simulink model "TV_2017_HIL"  (R2016a)
settings: Solver=ode1  StartTime=0.0  StopTime=600  FixedStep=0.001  RelTol=1e-3
PreLoadFcn:
  | HIL_parameters
values from neighbouring files (symbols this model uses):
  battery_voltage = single(530)    [HIL_parameters.m]    (also in HIL_parameters_2018.m; TV_2017_parameters.m; TV_2017_parameters_VD.m)
  car_params = Simulink_Car_params    [HIL_parameters.m]    (also in HIL_parameters_2018.m; TV_2017_parameters.m; TV_2017_parameters_VD.m)
  i_Diff = 16    [HIL_parameters.m]    (also in HIL_parameters_2018.m; TV_2017_parameters.m)
  Kp = 1    [HIL_parameters.m]    (also in HIL_parameters_2018.m; TV_2017_parameters.m; TV_2017_parameters_VD.m)
  motor_data = struct    [HIL_parameters.m]    (also in HIL_parameters_2018.m; TV_2017_parameters.m)
  settings = Simulink_Settings    [HIL_parameters.m]    (also in HIL_parameters_2018.m; TV_2017_parameters.m; TV_2017_parameters_VD.m)
  SpdC_BCC = 0    [HIL_parameters.m]    (also in HIL_parameters_2018.m; TV_2017_parameters.m; TV_2017_parameters_VD.m)
  Speed_Neg_sat = -21    [HIL_parameters.m]    (also in HIL_parameters_2018.m; TV_2017_parameters.m; TV_2017_parameters_VD.m)
  Speed_Pos_sat = 21    [HIL_parameters.m]    (also in HIL_parameters_2018.m; TV_2017_parameters.m; TV_2017_parameters_VD.m)
  SteeringAngleFL = [-23.80 -22.65 -21.50 -20.34 -19.18 -18.03 -16.86 -15.70 -14.53 -13.35 -12.18 -10.99 -9.80 -8.61 -7.40 -6.19 -4.97 -3.75 -2.51 -1.26 0 1.27 2.56 3.85 5.17 6.50 7.84 9.21 10.59 12.00 13.42 14.88 16.36 17.87 19.41 20.99 22.61 24.26 25.97 27.73 29.54]    [CarSetupAnalysis2018.m]    (also in HIL_parameters_2018.m; TV_2017_parameters.m; TV_2017_parameters_VD.m = [-24.129 -22.950 -21.772 -20.593 -19.413 -18.232 -17.050 -15)
  SteeringAngleFR = [-29.54 -27.73 -25.97 -24.26 -22.61 -20.99 -19.41 -17.87 -16.36 -14.88 -13.42 -12.00 -10.59 -9.21 -7.84 -6.50 -5.17 -3.85 -2.56 -1.27 0 1.26 2.51 3.75 4.97 6.19 7.40 8.61 9.80 10.99 12.18 13.35 14.53 15.70 16.86 18.03 19.18 20.34 21.50 22.65 23.80]    [CarSetupAnalysis2018.m]    (also in HIL_parameters_2018.m; TV_2017_parameters.m; TV_2017_parameters_VD.m = [-29.3050 -27.5340 -25.8140 -24.1410 -22.5110 -20.9180 -19.3)
  SteeringWhAngle = [-105 -99.75 -94.5 -89.25 -84 -78.75 -73.5 -68.25 -63 -57.75 -52.5 -47.25 -42 -36.75 -31.5 -26.25 -21.0 -15.75 -10.5 -5.25 0.0 5.25 10.50 15.75 21.00 26.25 31.50 36.75 42.00 47.25 52.50 57.75  63.00 68.25 73.50 78.75 84.00 89.25 94.50 99.75 105.00]    [TV_2017_parameters_VD.m]
  Tn_n = 0    [HIL_parameters.m]    (also in HIL_parameters_2018.m; TV_2017_parameters.m; TV_2017_parameters_VD.m)
  Use_Joystick = 1    [HIL_parameters.m]    (also in HIL_parameters_2018.m; TV_2017_parameters.m; TV_2017_parameters_VD.m)
undefined symbols (not defined in the file or in its folder): canChannel, TC_Decr_Gas, TC_Derivative, TC_Incr_Gas, TC_On, TC_Relay_Off, TC_Relay_On
libraries: CarMaker4SL x314, canmsglib x48, simulink_extras x48, simulink x41, canlib x39, powerlib_meascontrol x2, sldrtlib x1
(part 9 of 9)

== system TV_2017_HIL/CarMaker/IPG Vehicle3/CarAndTrailer/Forces/Tires/TireRR ==
  note: Insert your tire model here.
  Sync_In : Inport
  Load : Inport  Port=2
  vxtrans : Inport  Port=3
  vytrans : Inport  Port=4
  Rim_rotv : Inport  Port=5
  Rim_turnv : Inport  Port=6
  InclinAngle : Inport  Port=7
  muRoad : Inport  Port=8
  Ground{1..11} (11 alike) : Ground
  Terminator{,1..6,12} (8 alike) : Terminator
  Slp : Outport
  Alpha : Outport  Port=2
  TurnSlp : Outport  Port=3
  rBelt_eff : Outport  Port=4
  vBelt : Outport  Port=5
  LongFrc : Outport  Port=6
  SideFrc : Outport  Port=7
  LoadFrc : Outport  Port=8
  OverturnTrq : Outport  Port=9
  RollResist : Outport  Port=10
  AlignTrq : Outport  Port=11
  wires:
  Ground11/1 -> vBelt/1
  Ground10/1 -> rBelt_eff/1
  Ground9/1 -> TurnSlp/1
  Rim_turnv/1 -> Terminator6/1
  Sync_In/1 -> Terminator12/1
  Ground2/1 -> Alpha/1
  Ground3/1 -> LongFrc/1
  Ground4/1 -> SideFrc/1
  Ground5/1 -> OverturnTrq/1
  vxtrans/1 -> Terminator1/1
  vytrans/1 -> Terminator2/1
  Rim_rotv/1 -> Terminator3/1
  InclinAngle/1 -> Terminator4/1
  muRoad/1 -> Terminator5/1
  Load/1 -> Terminator/1
  Ground1/1 -> Slp/1
  Ground6/1 -> LoadFrc/1
  Ground7/1 -> RollResist/1
  Ground8/1 -> AlignTrq/1

== system TV_2017_HIL/CarMaker/IPG Vehicle3/CarAndTrailer/Forces/Vehicle Forces/Aero R18 prelim ==
  car Aero ApproachVel_1 x : Inport
  car Aero ApproachVel_1 y : Inport  Port=2
  car Aero ApproachVel_1 z : Inport  Port=3
  car Aero tau_1 : Inport  Port=4
  car Aero PoA_1 x : Inport  Port=5
  car Aero PoA_1 y : Inport  Port=6
  car Aero PoA_1 z : Inport  Port=7
  car Aero Frc_1 x : Inport  Port=8
  car Aero Frc_1 y : Inport  Port=9
  car Aero Frc_1 z : Inport  Port=10
  car Aero Trq_1 x : Inport  Port=11
  car Aero Trq_1 y : Inport  Port=12
  car Aero Trq_1 z : Inport  Port=13
  Coefficients : Subsystem
  Constant : Constant  Value=0
  Drag & DF : Scope  NumInputPorts=2
  MATLAB Function : MATLAB Function  TreatAsAtomicUnit=on
  Pitch moment : Scope
  Rad2Deg : simulink_extras/Transformations/Radians to Degrees
  Rad2Deg1 : simulink_extras/Transformations/Radians to Degrees
  Rad2Deg2 : simulink_extras/Transformations/Radians to Degrees
  Read CM Dict : CarMaker4SL/Read CM Dict  xname=Car.Roll  xsync=off
  Read CM Dict1 : CarMaker4SL/Read CM Dict  xname=Car.Pitch  xsync=off
  Read CM Dict2 : CarMaker4SL/Read CM Dict  xname=Car.TrackRadius  xsync=off
  Scope : Scope  Commented=on  NumInputPorts=2
  Terminator{,1..5} (6 alike) : Terminator
  Yaw moment : Scope
  car Aero ApproachVel_1 x_R18 : Outport
  car Aero ApproachVel_1 y_R18 : Outport  Port=2
  car Aero ApproachVel_1 z_R18 : Outport  Port=3
  car Aero tau_1_R18 : Outport  Port=4
  car Aero PoA_1 x_R18 : Outport  Port=5
  car Aero PoA_1 y_R18 : Outport  Port=6
  car Aero PoA_1 z_R18 : Outport  Port=7
  car Aero Frc_1 x_R18 : Outport  Port=8
  car Aero Frc_1 y_R18 : Outport  Port=9
  car Aero Frc_1 z_R18 : Outport  Port=10
  car Aero Trq_1 x_R18 : Outport  Port=11
  car Aero Trq_1 y_R18 : Outport  Port=12
  car Aero Trq_1 z_R18 : Outport  Port=13
  wires:
  Read CM Dict1/1 -> Rad2Deg1/1
  Read CM Dict/1 -> Rad2Deg/1
  car Aero PoA_1 x/1 -> car Aero PoA_1 x_R18/1
  car Aero PoA_1 y/1 -> car Aero PoA_1 y_R18/1
  car Aero PoA_1 z/1 -> car Aero PoA_1 z_R18/1
  Read CM Dict2/1 -> Scope/1, Coefficients/5(Radius)
  Rad2Deg1/1 -> Scope/2, Coefficients/2(Pitch)
  Rad2Deg/1 -> Coefficients/1(Roll)
  car Aero ApproachVel_1 x/1 -> MATLAB Function/1(Vx), car Aero ApproachVel_1 x_R18/1
  car Aero ApproachVel_1 y/1 -> car Aero ApproachVel_1 y_R18/1, MATLAB Function/2(Vy)
  car Aero ApproachVel_1 z/1 -> car Aero ApproachVel_1 z_R18/1
  car Aero tau_1/1 -> Rad2Deg2/1, car Aero tau_1_R18/1
  Coefficients/1(Coeffs) -> MATLAB Function/3(coeffs)
  MATLAB Function/4(Mx) -> car Aero Trq_1 x_R18/1
  MATLAB Function/1(Fx) -> Drag & DF/1, car Aero Frc_1 x_R18/1
  MATLAB Function/2(Fy) -> car Aero Frc_1 y_R18/1
  Constant/1 -> Coefficients/3(Rideheigth)
  car Aero Frc_1 x/1 -> Terminator/1
  car Aero Frc_1 y/1 -> Terminator1/1
  car Aero Frc_1 z/1 -> Terminator2/1
  car Aero Trq_1 x/1 -> Terminator3/1
  car Aero Trq_1 y/1 -> Terminator4/1
  car Aero Trq_1 z/1 -> Terminator5/1
  MATLAB Function/3(Fz) -> Drag & DF/2, car Aero Frc_1 z_R18/1
  MATLAB Function/5(My) -> Pitch moment/1, car Aero Trq_1 y_R18/1
  MATLAB Function/6(Mz) -> Yaw moment/1, car Aero Trq_1 z_R18/1
  Rad2Deg2/1 -> Coefficients/4(Yaw)

== system TV_2017_HIL/CarMaker/IPG Vehicle3/PowerTrain/Electric Powertrain/E-Gas // E-Motor/Electronic Gas Pedal RL ==
  TC_On : Inport
  VC.Gas : Inport  Port=2
  Define CM Dict : CarMaker4SL/Define CM Dict  xname=E_Gas_RL  xmono=off  xtype=Double4  xdvaplace=None  xnstates=0  xfirststate=0  xinitial=0
  Read CM Dict1 : CarMaker4SL/Read CM Dict  xname=E_Gas_RL  xsync=off
  Read CM Dict2 : CarMaker4SL/Read CM Dict  xname=Car.LongSlipRL  xsync=off
  Subsystem1 : Subsystem
  Switch : Switch
  Write CM Dict : CarMaker4SL/Write CM Dict  xname=E_Gas_RL  xsync=off
  Motor_Gas_RL : Outport
  wires:
  VC.Gas/1 -> Switch/3, Subsystem1/1(VC.Gas)
  Switch/1 -> Motor_Gas_RL/1
  TC_On/1 -> Switch/2
  Subsystem1/1(E_Gas) -> Write CM Dict/1, Switch/1
  Read CM Dict1/1 -> Subsystem1/2(E_Gas.)
  Read CM Dict2/1 -> Subsystem1/3(Car.LongSlip)

== system TV_2017_HIL/CarMaker/IPG Vehicle3/PowerTrain/Electric Powertrain/E-Gas // E-Motor/Electronic Gas Pedal RR ==
  TC_On : Inport
  VC.Gas : Inport  Port=2
  Define CM Dict : CarMaker4SL/Define CM Dict  xname=E_Gas_RR  xmono=off  xtype=Double4  xdvaplace=None  xnstates=0  xfirststate=0  xinitial=0
  Read CM Dict1 : CarMaker4SL/Read CM Dict  xname=E_Gas_RR  xsync=off
  Read CM Dict2 : CarMaker4SL/Read CM Dict  xname=Car.LongSlipRR  xsync=off
  Subsystem1 : Subsystem
  Switch : Switch
  Write CM Dict : CarMaker4SL/Write CM Dict  xname=E_Gas_RR  xsync=off
  Motor_Gas_RR : Outport
  wires:
  TC_On/1 -> Switch/2
  Switch/1 -> Motor_Gas_RR/1
  VC.Gas/1 -> Switch/3, Subsystem1/1(VC.Gas)
  Subsystem1/1(E_Gas) -> Write CM Dict/1, Switch/1
  Read CM Dict2/1 -> Subsystem1/3(Car.LongSlip)
  Read CM Dict1/1 -> Subsystem1/2(E_Gas.)

== system TV_2017_HIL/CarMaker/IPG Vehicle3/PowerTrain/Electric Powertrain/E-Gas // E-Motor/Rotation RL ==
  Gain : Gain  Gain=i_Diff
  Gain1 : Gain  Gain=60/(2*pi)
  Read CM Dict : CarMaker4SL/Read CM Dict  xname=Car.WheelSpd_RL  xsync=off
  Engine_rot_RL : Outport
  wires:
  Read CM Dict/1 -> Gain/1
  Gain/1 -> Gain1/1
  Gain1/1 -> Engine_rot_RL/1

== system TV_2017_HIL/CarMaker/IPG Vehicle3/PowerTrain/Electric Powertrain/E-Gas // E-Motor/Rotation RR ==
  Gain : Gain  Gain=i_Diff
  Gain1 : Gain  Gain=60/(2*pi)
  Read CM Dict : CarMaker4SL/Read CM Dict  xname=Car.WheelSpd_RR  xsync=off
  Engine_rot_RR : Outport
  wires:
  Gain1/1 -> Engine_rot_RR/1
  Gain/1 -> Gain1/1
  Read CM Dict/1 -> Gain/1

== system TV_2017_HIL/CarMaker/IPG Vehicle2/CarAndTrailer/Forces/Vehicle Forces/Aerodynamics R17/Coeff_x DRS Closed ==
  Roll : Inport
  Pitch : Inport  Port=2
  Rideheight : Inport  Port=3
  1-D Lookup Cd-pitch : Lookup_n-D  NumberOfTableDimensions=1  BreakpointsForDimension1=[-1,0,1]  Table=[1.31, 1.459, 1.41]  InternalRulePriority=Speed  RndMeth=Simplest  InputSameDT=on
  1-D Lookup Cl-pitch1 : Lookup_n-D  NumberOfTableDimensions=1  BreakpointsForDimension1=[-1,0,1]  Table=[2.77, 3.295, 3.43]  InternalRulePriority=Speed  RndMeth=Simplest  InputSameDT=on
  1-D Lookup Cl-pitch2 : Lookup_n-D  NumberOfTableDimensions=1  BreakpointsForDimension1=[-1,0,1]  Table=[-0.099, 0.03596, 0.212]  InternalRulePriority=Speed  RndMeth=Simplest  InputSameDT=on
  Bus Creator : BusCreator  Inputs=6
  Cd : Constant  Value=1.459
  Cl : Constant  Value=3.295
  Cpm : Constant  Value=0.03596
  Crm : Constant  Value=0
  Cs : Constant  Value=0
  Cym : Constant  Value=0
  Terminator{1..4,8} (5 alike) : Terminator
  Coeff_x : Outport
  wires:
  1-D Lookup Cl-pitch1/1 -> Bus Creator/3  "Cl"
  Cs/1 -> Bus Creator/2  "Cs"
  Cym/1 -> Bus Creator/6  "Cym"
  1-D Lookup Cl-pitch2/1 -> Bus Creator/5  "Cpm"
  Crm/1 -> Bus Creator/4  "Crm"
  Bus Creator/1 -> Coeff_x/1
  1-D Lookup Cd-pitch/1 -> Bus Creator/1  "Cd"
  Rideheight/1 -> Terminator3/1
  Pitch/1 -> 1-D Lookup Cl-pitch1/1, 1-D Lookup Cl-pitch2/1, 1-D Lookup Cd-pitch/1
  Roll/1 -> Terminator8/1
  Cd/1 -> Terminator1/1  "Cd"
  Cl/1 -> Terminator2/1  "Cl"
  Cpm/1 -> Terminator4/1  "Cpm"

== system TV_2017_HIL/CarMaker/IPG Vehicle2/CarAndTrailer/Forces/Vehicle Forces/Aerodynamics R17/Coeff_x DRS Open ==
  Roll : Inport
  Pitch : Inport  Port=2
  Rideheight : Inport  Port=3
  Bus Creator : BusCreator  Inputs=6
  Cd : Constant  Value=0.861
  Cl : Constant  Value=2.4376
  Cpm : Constant  Value=0.21301
  Crm : Constant  Value=0
  Cs : Constant  Value=0
  Cym : Constant  Value=0
  Terminator : Terminator
  Terminator1 : Terminator
  Terminator2 : Terminator
  Coeff_x : Outport
  wires:
  Cl/1 -> Bus Creator/3
  Cs/1 -> Bus Creator/2
  Cym/1 -> Bus Creator/6
  Cpm/1 -> Bus Creator/5
  Crm/1 -> Bus Creator/4
  Bus Creator/1 -> Coeff_x/1
  Pitch/1 -> Terminator1/1
  Roll/1 -> Terminator/1
  Cd/1 -> Bus Creator/1
  Rideheight/1 -> Terminator2/1

== system TV_2017_HIL/CarMaker/IPG Vehicle2/CarAndTrailer/Forces/Vehicle Forces/Aerodynamics R17/Coeff_y DRS Closed ==
  Roll : Inport
  Pitch : Inport  Port=2
  Rideheight : Inport  Port=3
  Bus Creator : BusCreator  Inputs=6
  Cd_y : Constant  Value=0
  Cl_y : Constant  Value=0
  Cpm_y : Constant  Value=0
  Crm_y : Constant  Value=0
  Cs_y : Constant  Value=0
  Cym_y : Constant  Value=0
  Terminator1 : Terminator
  Terminator2 : Terminator
  Terminator3 : Terminator
  Coeff_y : Outport
  wires:
  Cl_y/1 -> Bus Creator/3  "Cl_y"
  Cs_y/1 -> Bus Creator/2  "Cs_y"
  Cym_y/1 -> Bus Creator/6  "Cym_y"
  Cpm_y/1 -> Bus Creator/5  "Cpm_y"
  Crm_y/1 -> Bus Creator/4  "Crm_y"
  Bus Creator/1 -> Coeff_y/1
  Cd_y/1 -> Bus Creator/1  "Cd_y"
  Rideheight/1 -> Terminator3/1
  Pitch/1 -> Terminator1/1
  Roll/1 -> Terminator2/1

== system TV_2017_HIL/CarMaker/IPG Vehicle2/CarAndTrailer/Forces/Vehicle Forces/Aerodynamics R17/DRS Control ==
  Constant : Constant  Value=0
  DRS : Scope  Commented=on
  DRSactuation : MATLAB Function  TreatAsAtomicUnit=on
  Define CM Dict1 : CarMaker4SL/Define CM Dict  xname=DRS  xmono=off  xtype=Double  xdvaplace=None  xnstates=0  xfirststate=0  xinitial=0
  Enable/disable : Constant  Value=car_params.DRSenable
  Off Delay : powerlib_meascontrol/Logic/On Delay  DelayType=Off delay  delay=0.15  ic=1  Ts=0
  On Delay : powerlib_meascontrol/Logic/On Delay  DelayType=On delay  delay=0.15  ic=0  Ts=0
  Power : Scope  Commented=on
  Rad2DegConv7 : simulink_extras/Transformations/Radians to Degrees
  Read CM Dict : CarMaker4SL/Read CM Dict  xname=Power  xsync=off
  SteerAng : Scope  Commented=on
  SteerAngle : CarMaker4SL/Read CM Dict  xname=DM.Steer.Ang  xsync=off
  Switch : Switch  Criteria=u2 ~= 0
  Write CM Dict : CarMaker4SL/Write CM Dict  xname=DRS  xsync=off
  DRSopen : Outport
  wires:
  SteerAngle/1 -> Rad2DegConv7/1
  Switch/1 -> DRS/1, Write CM Dict/1, DRSopen/1  "DRSopen"
  Rad2DegConv7/1 -> SteerAng/1, DRSactuation/2(SteerAng)  "SteerAng"
  Read CM Dict/1 -> DRSactuation/1(P), Power/1  "Power"
  On Delay/1 -> Switch/1
  Off Delay/1 -> On Delay/1
  Constant/1 -> Switch/3
  Enable/disable/1 -> Switch/2
  DRSactuation/1(Status) -> Off Delay/1

== system TV_2017_HIL/CarMaker/IPG Vehicle2/CarAndTrailer/Forces/Vehicle Forces/Aerodynamics R17/RideheightEstimation ==
  note: Need to consider motion ratio?? rough estimate...
  Constant : Constant  Value=4
  Define CM Dict : CarMaker4SL/Define CM Dict  xname=RideHeight  xmono=off  xtype=Double  xdvaplace=None  xnstates=0  xfirststate=0  xinitial=0
  Divide : Product  Inputs=*/
  Initial length (mid pos) : Constant  Value=0.1746
  Scope : Scope
  SpringLegthrR : CarMaker4SL/Read CM Dict  xname=Car.SpringRR.l  xsync=off
  SpringLengthFL : CarMaker4SL/Read CM Dict  xname=Car.SpringFL.l  xsync=off
  SpringLengthFR : CarMaker4SL/Read CM Dict  xname=Car.SpringFR.l  xsync=off
  SpringLengthRL : CarMaker4SL/Read CM Dict  xname=Car.SpringRL.l  xsync=off
  Static height : Constant  Value=car_params.InitRideheight
  Subtract{,1..4} (5 alike) : Sum  Inputs=+-
  Sum : Sum  Inputs=|++++
  Write CM Dict : CarMaker4SL/Write CM Dict  xname=RideHeight  xsync=off
  Rideheight : Outport
  wires:
  SpringLegthrR/1 -> Subtract3/2
  Subtract1/1 -> Sum/2  "FR"
  Subtract/1 -> Sum/1  "FL"
  Initial length (mid pos)/1 -> Subtract/1, Subtract1/1, Subtract2/1, Subtract3/1
  SpringLengthRL/1 -> Subtract2/2
  SpringLengthFL/1 -> Subtract/2
  SpringLengthFR/1 -> Subtract1/2
  Subtract2/1 -> Sum/3  "RL"
  Subtract3/1 -> Sum/4  "RR"
  Sum/1 -> Divide/1
  Divide/1 -> Subtract4/2
  Constant/1 -> Divide/2
  Static height/1 -> Subtract4/1
  Subtract4/1 -> Write CM Dict/1, Scope/1, Rideheight/1

== system TV_2017_HIL/CarMaker/IPG Vehicle3/CarAndTrailer/Forces/Vehicle Forces/Aero R18 prelim/Coefficients ==
  Roll : Inport
  Pitch : Inport  Port=2
  Rideheigth : Inport  Port=3
  Yaw : Inport  Port=4
  Radius : Inport  Port=5
  1-D Lookup Pitch Cd : Lookup_n-D  NumberOfTableDimensions=1  BreakpointsForDimension1=[-1,0,1]  Table=[0.95*1.563,1.563,1.025*1.563]  ExtrapMethod=Clip  UseLastTableValue=on  InternalRulePriority=Speed  RndMeth=Simplest  InputSameDT=on
  1-D Lookup Pitch Cl : Lookup_n-D  NumberOfTableDimensions=1  BreakpointsForDimension1=[-1,0,1]  Table=[0.9*4.205,4.205,1.05*4.205]  ExtrapMethod=Clip  UseLastTableValue=on  InternalRulePriority=Speed  RndMeth=Simplest  InputSameDT=on
  1-D Lookup Pitch Cpm : Lookup_n-D  NumberOfTableDimensions=1  BreakpointsForDimension1=[-1,0,1]  Table=[-0.099, 0.03596, 0.212]  ExtrapMethod=Clip  UseLastTableValue=on  InternalRulePriority=Speed  RndMeth=Simplest  InputSameDT=on
  1-D Lookup Radii Cym : Lookup_n-D  NumberOfTableDimensions=1  BreakpointsForDimension1=[6,9.125,20,100]  Table=[-0.275,-0.175,-0.1,0]  ExtrapMethod=Clip  UseLastTableValue=on  InternalRulePriority=Speed  RndMeth=Simplest  InputSameDT=on
  "1-D Lookup Yaw, norm Cd" : Lookup_n-D  NumberOfTableDimensions=1  BreakpointsForDimension1=[-10,-5,0,5,10]  Table=[1.04,1.03,1.0,1.03,1.04]  ExtrapMethod=Clip  UseLastTableValue=on  InternalRulePriority=Speed  RndMeth=Simplest  InputSameDT=on
  "1-D Lookup Yaw, norm Cl" : Lookup_n-D  NumberOfTableDimensions=1  BreakpointsForDimension1=[-10,-5,0,5,10]  Table=[0.93,0.97,1.0,0.97,0.93]  ExtrapMethod=Clip  UseLastTableValue=on  InternalRulePriority=Speed  RndMeth=Simplest  InputSameDT=on
  Abs : Abs
  BusCreator : BusCreator  Inputs=6
  Crm : Constant  Value=0
  Cs : Constant  Value=0
  Cym factor : Constant  Value=0.5
  Product : Product
  Product1 : Product
  Product2 : Product  Inputs=3
  Sign : Signum
  Terminator : Terminator
  Terminator2 : Terminator
  Coeffs : Outport
  wires:
  Rideheigth/1 -> Terminator/1
  Radius/1 -> Sign/1, Abs/1
  Yaw/1 -> "1-D Lookup Yaw, norm Cl"/1, "1-D Lookup Yaw, norm Cd"/1
  Roll/1 -> Terminator2/1
  Pitch/1 -> 1-D Lookup Pitch Cd/1, 1-D Lookup Pitch Cl/1, 1-D Lookup Pitch Cpm/1
  Product/1 -> BusCreator/1  "Cd"
  Cs/1 -> BusCreator/2  "Cs"
  Product1/1 -> BusCreator/3  "Cl"
  Crm/1 -> BusCreator/4  "Crm"
  1-D Lookup Pitch Cpm/1 -> BusCreator/5  "Cpm"
  BusCreator/1 -> Coeffs/1  "coeffs"
  1-D Lookup Pitch Cd/1 -> Product/1
  1-D Lookup Pitch Cl/1 -> Product1/1
  "1-D Lookup Yaw, norm Cd"/1 -> Product/2
  "1-D Lookup Yaw, norm Cl"/1 -> Product1/2
  Abs/1 -> 1-D Lookup Radii Cym/1
  1-D Lookup Radii Cym/1 -> Product2/1  "Cym"
  Product2/1 -> BusCreator/6  "Cym"
  Cym factor/1 -> Product2/2
  Sign/1 -> Product2/3

== system TV_2017_HIL/CarMaker/IPG Vehicle3/PowerTrain/Electric Powertrain/E-Gas // E-Motor/Electronic Gas Pedal RL/Subsystem1 ==
  VC.Gas : Inport
  E_Gas. : Inport  Port=2
  Car.LongSlip : Inport  Port=3
  Add : Sum
  Compare To Constant : simulink/Logic and Bit Operations/Compare To Constant  relop=>  const=TC_Derivative  OutDataTypeStr=uint8  ZeroCross=off
  Derivative : Derivative
  Fcn : Fcn  Expr=u >0.05
  Fcn1 : Fcn  Expr=u+TC_Incr_Gas
  Fcn2 : Fcn  Expr=u-TC_Decr_Gas
  Multiport Switch : MultiPortSwitch  DataPortOrder=Zero-based contiguous  zeroidx=on
  Relational Operator : RelationalOperator  Operator=<=
  Relay : Relay  OnSwitchValue=TC_Relay_On  OffSwitchValue=TC_Relay_Off
  S-R Flip-Flop : simulink_extras/Flip Flops/S-R Flip-Flop  initial_condition=0
  Saturation : Saturate  UpperLimit=1  LowerLimit=0
  Saturation1 : Saturate  UpperLimit=1  LowerLimit=0
  Switch : Switch  Criteria=u2 > Threshold
  Terminator : Terminator
  E_Gas : Outport
  wires:
  Car.LongSlip/1 -> Relay/1, Derivative/1, Fcn/1
  Relay/1 -> Add/1
  Derivative/1 -> Compare To Constant/1
  Compare To Constant/1 -> Add/2
  Add/1 -> Multiport Switch/1
  Multiport Switch/1 -> E_Gas/1
  VC.Gas/1 -> Relational Operator/1, [A]
  E_Gas./1 -> Relational Operator/2, Fcn1/1, Fcn2/1, Multiport Switch/3
  S-R Flip-Flop/2 -> Terminator/1
  S-R Flip-Flop/1 -> Switch/2
  Switch/1 -> Multiport Switch/2
  Fcn/1 -> S-R Flip-Flop/1
  Relational Operator/1 -> S-R Flip-Flop/2
  Fcn1/1 -> Saturation1/1
  Saturation1/1 -> Switch/1
  Fcn2/1 -> Saturation/1
  Saturation/1 -> Multiport Switch/4
  [A] -> Switch/3

== system TV_2017_HIL/CarMaker/IPG Vehicle3/PowerTrain/Electric Powertrain/E-Gas // E-Motor/Electronic Gas Pedal RR/Subsystem1 ==
  VC.Gas : Inport
  E_Gas. : Inport  Port=2
  Car.LongSlip : Inport  Port=3
  Add : Sum
  Compare To Constant : simulink/Logic and Bit Operations/Compare To Constant  relop=>  const=TC_Derivative  OutDataTypeStr=uint8  ZeroCross=off
  Derivative : Derivative
  Fcn : Fcn  Expr=u >0.05
  Fcn1 : Fcn  Expr=u+TC_Incr_Gas
  Fcn2 : Fcn  Expr=u-TC_Decr_Gas
  Multiport Switch : MultiPortSwitch  DataPortOrder=Zero-based contiguous  zeroidx=on
  Relational Operator : RelationalOperator  Operator=<=  InputSameDT=on
  Relay : Relay  OnSwitchValue=TC_Relay_On  OffSwitchValue=TC_Relay_Off
  S-R Flip-Flop : simulink_extras/Flip Flops/S-R Flip-Flop  initial_condition=0
  Saturation : Saturate  UpperLimit=1  LowerLimit=0
  Saturation1 : Saturate  UpperLimit=1  LowerLimit=0
  Switch : Switch  Criteria=u2 > Threshold
  Terminator : Terminator
  E_Gas : Outport
  wires:
  Car.LongSlip/1 -> Relay/1, Derivative/1, Fcn/1
  Relay/1 -> Add/1
  Derivative/1 -> Compare To Constant/1
  Compare To Constant/1 -> Add/2
  Add/1 -> Multiport Switch/1
  Multiport Switch/1 -> E_Gas/1
  VC.Gas/1 -> Relational Operator/1, [A]
  E_Gas./1 -> Relational Operator/2, Fcn1/1, Fcn2/1, Multiport Switch/3
  S-R Flip-Flop/2 -> Terminator/1
  S-R Flip-Flop/1 -> Switch/2
  Switch/1 -> Multiport Switch/2
  Fcn/1 -> S-R Flip-Flop/1
  Relational Operator/1 -> S-R Flip-Flop/2
  Fcn1/1 -> Saturation1/1
  Saturation1/1 -> Switch/1
  Fcn2/1 -> Saturation/1
  Saturation/1 -> Multiport Switch/4
  [A] -> Switch/3

== matlab function TV_2017_HIL/CarMaker/IPG Vehicle3/CarAndTrailer/Forces/Vehicle Forces/Aero R18 prelim/MATLAB Function ==
  data: Fx output; Vx input; Vy input; Fy output; Fz output; Mx output; My output; Mz output; coeffs input; car_params parameter
function [Fx,Fy,Fz,Mx,My,Mz] = AeroForceCalc(Vx,Vy,coeffs, car_params)
rho = double(car_params.AirDens);
A = double(car_params.aero_ref_area);
l = double(car_params.l);                % Wheelbase

V = sqrt(Vx^2+Vy^2);

Cd = coeffs(1);
Cs = coeffs(2);
Cl = coeffs(3);
Crm = coeffs(4);
Cpm = coeffs(5);
Cym = coeffs(6);

Fx = -(rho/2)*Cd*A*V^2;     % Drag force
Fy = (rho/2)*Cs*A*V^2;     % Side force
Fz = -(rho/2)*Cl*A*V^2;     % Downforce
Mx = (rho/2)*Crm*l*A*V^2;   % Roll moment
My = (rho/2)*Cpm*l*A*V^2;   % Pitch moment
Mz = (rho/2)*Cym*l*A*V^2;   % Yaw moment


end

== matlab function TV_2017_HIL/CarMaker/Function-Call Subsystem4/AMK Inverter Setpoints from ECU/MATLAB Function1 ==
  data: w_set_f output; w_set_16 input; trq_pos_16 input; trq_pos_f output; trq_neg_16 input; trq_neg_f output; settings parameter
function [w_set_f, trq_pos_f, trq_neg_f ] = fcn( w_set_16,trq_pos_16, trq_neg_16, settings)
%#codegen

Sf = 0.0098;%setpoint to inverters is given as  0.1% of 9.8(nominal torque)

trq_pos_f = double( trq_pos_16*Sf);
trq_neg_f = double( trq_neg_16*Sf);
w_set_f = double( w_set_16);

== matlab function TV_2017_HIL/CarMaker/Function-Call Subsystem4/AMK Inverter Setpoints from ECU/MATLAB Function2 ==
  data: w_set_f output; w_set_16 input; trq_pos_16 input; trq_pos_f output; trq_neg_16 input; trq_neg_f output; settings parameter
function [w_set_f, trq_pos_f, trq_neg_f ] = fcn( w_set_16,trq_pos_16, trq_neg_16, settings)
%#codegen

Sf = 0.0098;%setpoint to inverters is given as  0.1% of 9.8(nominal torque)

trq_pos_f = double( trq_pos_16*Sf);
trq_neg_f = double( trq_neg_16*Sf);
w_set_f = double( w_set_16);

== matlab function TV_2017_HIL/CarMaker/Function-Call Subsystem4/AMK Inverter Setpoints from ECU/MATLAB Function3 ==
  data: w_set_f output; w_set_16 input; trq_pos_16 input; trq_pos_f output; trq_neg_16 input; trq_neg_f output; settings parameter
function [w_set_f, trq_pos_f, trq_neg_f ] = fcn( w_set_16,trq_pos_16, trq_neg_16, settings)
%#codegen

Sf = 0.0098;%setpoint to inverters is given as  0.1% of 9.8(nominal torque)

trq_pos_f = double( trq_pos_16*Sf);
trq_neg_f = double( trq_neg_16*Sf);
w_set_f = double( w_set_16);

== matlab function TV_2017_HIL/CarMaker/ECU input Sensors /estimated "Measured Power" based on Torque, RPM and datasheet IRL this is measured/MATLAB Function ==
  data: RPM_FL_IN input; RPM_FR_IN input; RPM_RL_IN input; RPM_RR_IN input; Pm_FL output; T input; T_FL output; RPM_FL output; Pm_FR output; T_FR output; RPM_FR output; Pm_RL output; T_RL output; RPM_RL output; Pm_RR output; T_RR output; RPM_RR output
function [Pm_FL, T_FL, RPM_FL,Pm_FR, T_FR, RPM_FR,Pm_RL, T_RL,...
          RPM_RL,Pm_RR, T_RR, RPM_RR] = powerMeasurement(RPM_FL_IN, RPM_FR_IN,RPM_RL_IN,RPM_RR_IN, T)
%#codegen

%Conversion from RPM to rad/s
c = single(2*pi/60);

T_FL = T.FL;
T_FR = T.FR;
T_RL = T.RL;
T_RR = T.RR;

RPM_FL = RPM_FL_IN;
RPM_FR = RPM_FR_IN;
RPM_RL = RPM_RL_IN;
RPM_RR = RPM_RR_IN;


Pm_FL = RPM_FL*c*T.FL;
Pm_FR = RPM_FR*c*T.FR;
Pm_RL = RPM_RL*c*T.RL;
Pm_RR = RPM_RR*c*T.RR;

== matlab function TV_2017_HIL/CarMaker/Function-Call Subsystem4/AMK Inverter Setpoints from ECU/MATLAB Function ==
  data: w_set_f output; w_set_16 input; trq_pos_16 input; trq_pos_f output; trq_neg_16 input; trq_neg_f output; settings parameter
function [w_set_f, trq_pos_f, trq_neg_f ] = fcn( w_set_16,trq_pos_16, trq_neg_16, settings)
%#codegen
Sf = 0.0098; %setpoint to inverters is given as  0.1% of 9.8(nominal torque)

trq_pos_f = double( trq_pos_16*Sf);
trq_neg_f = double( trq_neg_16*Sf);
w_set_f = double( w_set_16);

== matlab function TV_2017_HIL/CarMaker/IPG Vehicle2/CarAndTrailer/Forces/Vehicle Forces/Aerodynamics R17/MATLAB Function ==
  data: Coeff_x input; Coeff_y input; Fx output; Vx input; Vy input; Fy output; Fz output; Mx output; My output; Mz output; car_params parameter
function [Fx,Fy,Fz,Mx,My,Mz] = AeroForceCalc(Coeff_x, Coeff_y,Vx,Vy,car_params)
rho = double(car_params.AirDens);
A = double(car_params.aero_ref_area);
l = double(car_params.l);                   % Wheelbase

Cd_x = Coeff_x(1);
Cs_x = Coeff_x(2);
Cl_x = Coeff_x(3);
Crm_x = Coeff_x(4);
Cpm_x = Coeff_x(5);
Cym_x = Coeff_x(6);

Cd_y = Coeff_y(1);
Cs_y = Coeff_y(2);
Cl_y = Coeff_y(3);
Crm_y = Coeff_y(4);
Cpm_y = Coeff_y(5);
Cym_y = Coeff_y(6);

Fx = -(rho/2)*Cd_x*A*Vx^2   - (rho/2)*Cd_y*A*Vy^2;      % Drag force
Fy = (rho/2)*Cs_x*A*Vx^2    + (rho/2)*Cs_y*A*Vy^2;      % Side force
Fz = -(rho/2)*Cl_x*A*Vx^2   - (rho/2)*Cl_y*A*Vy^2;      % Downforce
Mx = (rho/2)*Crm_x*l*A*Vx^2 + (rho/2)*Crm_y*l*A*Vy^2;   % Roll moment
My = (rho/2)*Cpm_x*l*A*Vx^2 + (rho/2)*Cpm_y*l*A*Vy^2;   % Pitch moment
Mz = (rho/2)*Cym_x*l*A*Vx^2 + (rho/2)*Cym_y*l*A*Vy^2;   % Yaw moment
end

== matlab function TV_2017_HIL/CarMaker/VehicleControl2/CreateBus VhclCtrl/Add KERS ==
  data: brake_pedal input; KERS_pos output; brake_pos output
function [KERS_pos, brake_pos] = fcn(brake_pedal)
%#codegen

% 0-0.5 = KERS , 0.5-1.0 = 0-1 brake
    KERS_pos = single(0);
    brake_pos = 0;
    if brake_pedal >= 0 & brake_pedal <=  0.5
        KERS_pos = single(2*brake_pedal);
        brake_pos = 0;
    else
        KERS_pos = single(1);
        brake_pos = 2*(brake_pedal -0.5);
    end
    
%     if brake_pedal >= 0 & brake_pedal <=  1.0001
%         KERS_pos = single(brake_pedal);
%         brake_pos = 0;
%     else
%         KERS_pos = single(1);
%         brake_pos = 2*(brake_pedal -0.5);
%     end


end

== matlab function TV_2017_HIL/CarMaker/IPG Vehicle2/CarAndTrailer/Forces/Vehicle Forces/Aerodynamics R17/DRS Control/DRSactuation ==
  data: P input; Status output; SteerAng input; car_params parameter
function Status = DRSactuation(P,SteerAng,car_params)
functionality = car_params.DRSenable;
P_min = car_params.DRS_Pmin;
Steer_max = car_params.DRS_SteerMax;
SteerAng = abs(SteerAng);
if functionality == 1
    if (P>=P_min && SteerAng<=Steer_max) 
        Status = single(1);
    else
        Status = single(0);
    end
elseif functionality == 2
    Status = single(1);
else
    Status = single(0);
end

== matlab function TV_2017_HIL/CarMaker/Debug Information /Vehicle dynamics analysis JMH/MATLAB Function1 ==
  data: Force input; MM output; Moment input; car_params parameter
function MM = MagicMumber(Force,Moment,car_params)
WB = car_params.l;              % Wheelbase
Lf = 2.03-car_params.AeroRefX;  % Distance from aero referance to front axle
Fz = Force(3);                  % aerodynamic lift
PM = Moment(2);                 % aerodynamic pitch moment
Fr = (-PM-Fz.*Lf)./WB;           % aerodynamic load rear axle
Ff = -Fz-Fr;                    % aerodynamic load front axle
MM = Fr./(Ff+Fr);               % front-rear aerodynamic balance metric
end

== matlab function TV_2017_HIL/CarMaker/Debug Information /Vehicle dynamics analysis JMH/MATLAB Function ==
  data: V input; OM_transient output; Delta input; Ay input; YawRate input; car_params parameter; OM_steadystate output
function [OM_transient,OM_steadystate] = OversteerMetric(V,Delta,Ay,YawRate,car_params)
W = car_params.l;
avgDelta = mean(Delta).*pi/180;     
AKR = V.*tan(avgDelta)./W;
OM_transient = YawRate-AKR;
OM_steadystate = (Ay.*W)./V.^2-avgDelta;
end

== matlab function TV_2017_HIL/CarMaker/VehicleControl2/CreateBus VhclCtrl/RacingwheelInterface/Add KERS ==
  data: brake_pedal input; KERS_pos output; brake_pos output
function [KERS_pos, brake_pos] = fcn(brake_pedal)
%#codegen

% 0-0.5 = KERS , 0.5-1.0 = 0-1 brake
    KERS_pos = single(0);
    brake_pos = 0;
    if (brake_pedal > 0) && (brake_pedal <  0.5)
        KERS_pos = single(2*brake_pedal);
        brake_pos = 0;
    else
        KERS_pos = single(1);
        brake_pos = 2*(brake_pedal -0.5);
    end
    
%     if brake_pedal >= 0 & brake_pedal <=  1.0001
%         KERS_pos = single(brake_pedal);
%         brake_pos = 0;
%     else
%         KERS_pos = single(1);
%         brake_pos = 2*(brake_pedal -0.5);
%     end


end

== matlab function TV_2017_HIL/CarMaker/Debug Information /Fz_Estimation/FzEstDamper ==
  data: sensors input Bus: SensorInputs; Fz_damp_FL input; Fz_damp_FR input; Fz_damper_est output Bus: normalForces; Fz_damp_RL input; Fz_damp_RR input; car_params parameter; alfa_r output
function [Fz_damper_est, alfa_r] =  FzEstDamp(sensors, Fz_damp_FL, Fz_damp_FR, Fz_damp_RL, Fz_damp_RR, car_params)
%#codegen

Ks_front    = car_params.spring_constant_front;
Ks_rear     = car_params.spring_constant_rear;

 

preload_front = car_params.preload_front_mm;
preload_rear = car_params.preload_rear_mm;

unsprung = car_params.unsprung_mass_per_wheel_newton;

%esimate forces from spring and damper

Fz_damper_est.FL = Ks_front*sensors.damper_pos_FL + Fz_damp_FL;% 
Fz_damper_est.FR = Ks_front*sensors.damper_pos_FR + Fz_damp_FR;% 
Fz_damper_est.RL = Ks_rear*sensors.damper_pos_RL + Fz_damp_RL;% 
Fz_damper_est.RR = Ks_rear*sensors.damper_pos_RR + Fz_damp_RR;% 

alfa_r = (Fz_damper_est.RL + Fz_damper_est.RR) / (Fz_damper_est.FL + Fz_damper_est.FR + Fz_damper_est.RL + Fz_damper_est.RR);

%add unsprung mass to Fz estimate only when spring is loaded
add_unsprung_threshold = 10;
if (Fz_damper_est.FL>add_unsprung_threshold)
    Fz_damper_est.FL = Fz_damper_est.FL + unsprung; 
end
if (Fz_damper_est.FR>add_unsprung_threshold)
    Fz_damper_est.FR = Fz_damper_est.FR + unsprung; 
end
if (Fz_damper_est.RL>add_unsprung_threshold)
    Fz_damper_est.RL = Fz_damper_est.RL + unsprung; 
end
if (Fz_damper_est.RR>add_unsprung_threshold)
    Fz_damper_est.RR = Fz_damper_est.RR + unsprung; 
end


end

== matlab function TV_2017_HIL/CarMaker/Debug Information /Fz_Estimation/FzEstDamper 2016 ==
  data: sensors input Bus: SensorInputs; Fz_damp_FL input; Fz_damp_FR input; Fz_damper_est output Bus: normalForces; Fz_damp_RL input; Fz_damp_RR input; car_params parameter; alfa_r output
function [Fz_damper_est, alfa_r] =  FzEstDamp(sensors, Fz_damp_FL, Fz_damp_FR, Fz_damp_RL, Fz_damp_RR, car_params)
%#codegen

Ks_front    = car_params.spring_constant_front;
Ks_rear     = car_params.spring_constant_rear;

MR_front    = car_params.motion_ratio_front;
MR_rear     = car_params.motion_ratio_rear;     

preload_front = car_params.preload_front_mm;
preload_rear = car_params.preload_rear_mm;

%unsprung = car_params.unsprung_mass_per_wheel_newton;
% 0 - 1 mm, Go from 0 to neutral Fz
FL_scaling = single(min(sensors.damper_pos_FL, single(1)));
FR_scaling = single(min(sensors.damper_pos_FR, single(1)));
RL_scaling = single(min(sensors.damper_pos_RL, single(1)));
RR_scaling = single(min(sensors.damper_pos_RR, single(1)));

% Fz_damper_est.FL = (Ks_front*(sensors.damper_pos_FL + preload_front) + Fz_damp_FL)*MR_front + unsprung;
% Fz_damper_est.FR = (Ks_front*(sensors.damper_pos_FR + preload_front) + Fz_damp_FR)*MR_front + unsprung;
% Fz_damper_est.RL = (Ks_rear*(sensors.damper_pos_RL  + preload_rear)  + Fz_damp_RL)*MR_rear  + unsprung;
% Fz_damper_est.RR = (Ks_rear*(sensors.damper_pos_RR  + preload_rear)  + Fz_damp_RR)*MR_rear  + unsprung;

Fz_damper_est.FL = Ks_front*sensors.damper_pos_FL + Fz_damp_FL + (preload_front*Ks_front)*FL_scaling;
Fz_damper_est.FR = Ks_front*sensors.damper_pos_FR + Fz_damp_FR + (preload_front*Ks_front)*FR_scaling;
Fz_damper_est.RL = Ks_rear*sensors.damper_pos_RL + Fz_damp_RL + (preload_rear*Ks_rear)*RL_scaling;
Fz_damper_est.RR = Ks_rear*sensors.damper_pos_RR + Fz_damp_RR + (preload_rear*Ks_rear)*RR_scaling;

alfa_r = (Fz_damper_est.RL + Fz_damper_est.RR) / (Fz_damper_est.FL + Fz_damper_est.FR + Fz_damper_est.RL + Fz_damper_est.RR);
end

== matlab function TV_2017_HIL/CarMaker/Debug Information /Fz_Estimation/FzEstLoadTransfer ==
  data: Fz_loadTransfer_est output Bus: normalForces; sensor input Bus: SensorInputs; car_params parameter; vx input
function Fz_loadTransfer_est  = FzEstLoadTransfer(sensor,car_params,vx)
%#codegen




mv = car_params.car_mass + car_params.driver_mass; % Total mass( driver + car) X
l  = car_params.l; %Wheel base X
lr = car_params.l_r; % X
lf = car_params.l_f;% X

ef = car_params.t_f*2; % Front track X
er = car_params.t_r*2; % Rear track X


hc = car_params.CoG_height; % X
g = 9.81; % X
air_density = single(1.2);

Fz_loadTransfer_est.FL = single(0);%(0.5*mv*(lr*g/l - hc*sensor.ax/l) - mv*(lr*g/l - hc*sensor.ax/l)*hc*sensor.ay/(ef*g))  + (vx^2 * car_params.aero_ref_area* car_params.aero_lift_coeff*air_density)/8;
Fz_loadTransfer_est.FR = single(0);%(0.5*mv*(lr*g/l - hc*sensor.ax/l) + mv*(lr*g/l - hc*sensor.ax/l)*hc*sensor.ay/(ef*g))  + (vx^2 * car_params.aero_ref_area* car_params.aero_lift_coeff*air_density)/8;
Fz_loadTransfer_est.RL = single(0);%(0.5*mv*(lf*g/l + hc*sensor.ax/l) - mv*(lf*g/l + hc*sensor.ax/l)*hc*sensor.ay/(er*g))  + (vx^2 * car_params.aero_ref_area* car_params.aero_lift_coeff*air_density)/8;
Fz_loadTransfer_est.RR = single(0);%(0.5*mv*(lf*g/l + hc*sensor.ax/l) + mv*(lf*g/l + hc*sensor.ax/l)*hc*sensor.ay/(er*g))  + (vx^2 * car_params.aero_ref_area* car_params.aero_lift_coeff*air_density)/8;

end

== matlab function TV_2017_HIL/CarMaker/Debug Information /Subsystem/MATLAB Function ==
  data: RPM_FL_IN input; RPM_FR_IN input; RPM_RL_IN input; RPM_RR_IN input; Pm_FL output; T input; T_FL output; RPM_FL output; Pm_FR output; T_FR output; RPM_FR output; Pm_RL output; T_RL output; RPM_RL output; Pm_RR output; T_RR output; RPM_RR output
function [Pm_FL, T_FL, RPM_FL,Pm_FR, T_FR, RPM_FR,Pm_RL, T_RL,...
          RPM_RL,Pm_RR, T_RR, RPM_RR] = powerMeasurement(RPM_FL_IN, RPM_FR_IN,RPM_RL_IN,RPM_RR_IN, T)
%#codegen

%Conversion from RPM to rad/s
c = single(2*pi/60);

T_FL = T.FL;
T_FR = T.FR;
T_RL = T.RL;
T_RR = T.RR;

RPM_FL = RPM_FL_IN;
RPM_FR = RPM_FR_IN;
RPM_RL = RPM_RL_IN;
RPM_RR = RPM_RR_IN;


Pm_FL = RPM_FL*c*T.FL;
Pm_FR = RPM_FR*c*T.FR;
Pm_RL = RPM_RL*c*T.RL;
Pm_RR = RPM_RR*c*T.RR;

== matlab function TV_2017_HIL/CarMaker/Debug Information /SA calculation/Slip angle calc ==
  data: wheel_ang_left input; wheel_ang_right input; SA output Bus: SR; sensor input; car_params parameter
function SA  = slipRatioCalculation(wheel_ang_left,wheel_ang_right,sensor,car_params)
%#codegen
l_f = car_params.l_f;
t_f = car_params.t_f;   % why does *.7 help?
l_r = car_params.l_r;
t_r = car_params.t_r;
delta_left = wheel_ang_left; %sensor.steering_wheel_angle/4;
delta_right = wheel_ang_right; %sensor.steering_wheel_angle/4; % 
v_v_x = sensor.V_x_INS;
v_v_y = sensor.V_y_INS;
gamma_der = sensor.yawRate;
arm_len_front = sqrt(l_f^2+t_f^2);
arm_len_rear = sqrt(l_r^2+t_r^2);
corr_ang = -0.1*(2*pi/180)*0;

phi_FL =  atan(l_f/t_f);
phi_FR =  atan(l_f/t_f);
phi_RL =  atan(l_r/t_r);
phi_RR =  atan(l_r/t_r);

%tire frame  = vehicle speed adjusted for steer angle + decompsed
%contribution from yaw rate

%______________FL____________"intuitive" version calc independet wheel valocity in own frame_____________
v_x_FL =   cos(delta_left) * v_v_x  + sin(delta_left)  *  v_v_y   -  cos(delta_left)*t_f*gamma_der;
v_y_FL =  -sin(delta_left) * v_v_x  + cos(delta_left)  *  v_v_y   +  cos(delta_left)*l_f*gamma_der;   
% %______________FR_____________
v_x_FR =   cos(delta_right) * v_v_x + sin(delta_right) *  v_v_y   +  cos(delta_right)*t_f*gamma_der;  
v_y_FR =  -sin(delta_right) * v_v_x + cos(delta_right) *  v_v_y   +  cos(delta_right)*l_f*gamma_der;  
% %______________RL_____________
v_x_RL = v_v_x - t_r*gamma_der;
v_y_RL = v_v_y - l_r*gamma_der;
% %______________RR_____________
v_x_RR = v_v_x + t_r*gamma_der;
v_y_RR = v_v_y - l_r*gamma_der;




% direct method
SA.FL =  -single(   delta_left   -  atan(  (v_v_y  +  l_f * gamma_der) / abs(v_v_x  -  t_f*gamma_der) )   );
SA.FR =  -single(   delta_right  -  atan(  (v_v_y  +  l_f * gamma_der) / abs(v_v_x  +  t_f*gamma_der) )   );
SA.RL =  -single(                -  atan(  (v_v_y  -  l_r * gamma_der) / abs(v_v_x  -  t_r*gamma_der) )   );
SA.RR =  -single(                -  atan(  (v_v_y  -  l_r * gamma_der) / abs(v_v_x  +  t_r*gamma_der) )   );

% Using velocity compensated for yaw rate at each wheel hub
% SA.FL =   single(   atan(  v_y_FL / abs(v_x_FL) )   );
% SA.FR =   single(   atan(  v_y_FR / abs(v_x_FR) )   );
% SA.RL =   single(   atan(  v_y_RL / abs(v_x_RL) )   );
% SA.RR =   single(   atan(  v_y_RR / abs(v_x_RR) )   );
end
